simulink model "e2eDRL_ACC"  (R2023a)
settings: Solver=FixedStepAuto  StartTime=0.0  StopTime=200  FixedStep=0.1  RelTol=1e-3
values from neighbouring files (symbols this model uses):
  ap_maxmin = -3 + (0-(-4))*rand()    [Reset.m]
  beh = bernoulli_sample(prob_accp)    [Reset.m]
  dt = 0 + (2-0)*rand()    [Reset.m]    (also in Speed_replan.m = ds/v_backward(N+1-k))
  t1 = 5 + (100-5)*rand()    [Reset.m]
  Ts = 0.1    [Reset.m]
  v0_ego = 100/3.6    (= 27.7777777778)    [Reset.m]
  v0_lead = lower_bound_v0 + (upper_bound_v0-lower_bound_v0)*rand()    [Reset.m]
  v_des = sample_integer_interval(20,60,10)/3.6    [Reset.m]
  x0_ego = 0    [Reset.m]
  x0_lead = max(min(t_gap*v0_ego+D_default+5*randn(),80),15)    [Reset.m]
libraries: simulink x4
settings Model: Creator=The MathWorks, Inc.  LastModifiedBy=Administrator
settings SolverCC: AlgebraicLoopSolver=TrustRegion
settings DataIOCC: ReturnWorkspaceOutputs=off
settings DebuggingCC: UnconnectedInputMsg=warning  UnconnectedOutputMsg=warning  UnconnectedLineMsg=warning  ArithmeticOperatorsInVariantConditions=warning
settings ModelReferenceCC: EnableRefExpFcnMdlSchedulingChecks=on
settings SFSimCC: SimUseLocalCustomCode=off
settings RTWCC: RTWUseLocalCustomCode=off  DLArmComputeVersion=19.05
settings CodeAppCC: StateflowObjectComments=on

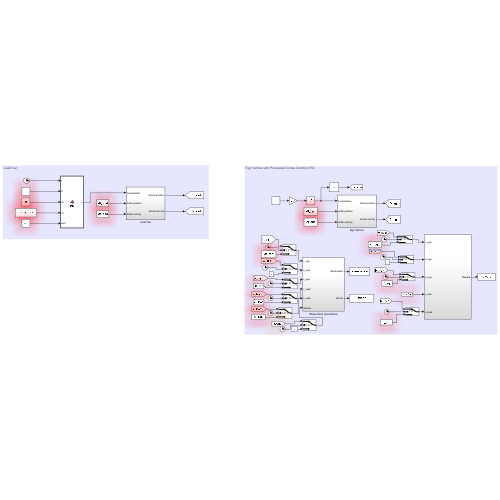
[thumbnail: Simulink's stored preview of the top-level diagram]
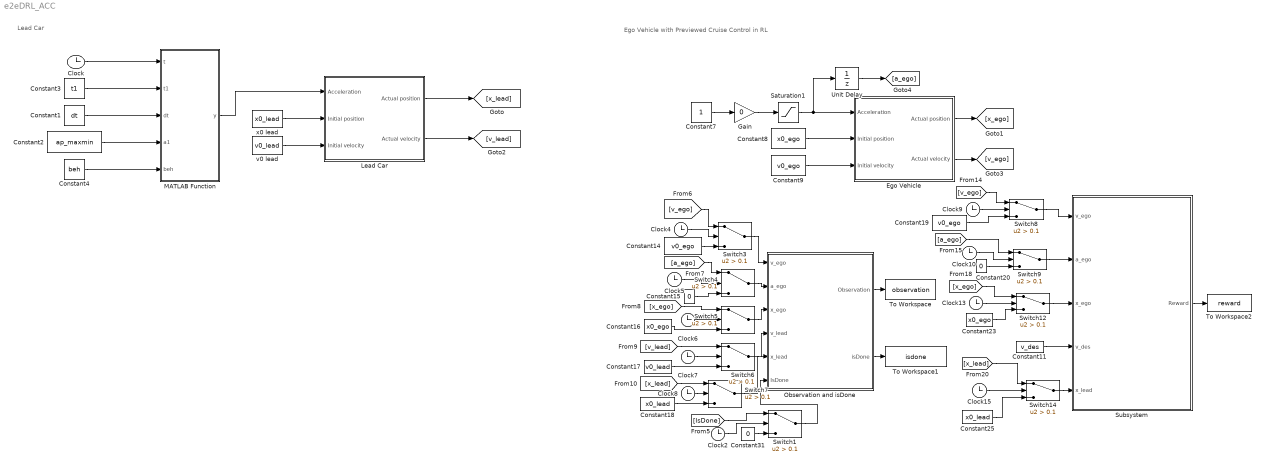
== system e2eDRL_ACC ==
  note: Lead Car
  note: Ego Vehicle with Previewed Cruise Control in RL
  Clock{,2,4..10,13,15} (11 alike) : Clock
  Constant1 : Constant  Value=dt  SampleTime=Ts
  Constant11 : Constant  Value=v_des  SampleTime=Ts
  Constant14 : Constant  Value=v0_ego  SampleTime=Ts
  Constant15 : Constant  Value=0
  Constant16 : Constant  Value=x0_ego  SampleTime=Ts
  Constant17 : Constant  Value=v0_lead  SampleTime=Ts
  Constant18 : Constant  Value=x0_lead  SampleTime=Ts
  Constant19 : Constant  Value=v0_ego  SampleTime=Ts
  Constant2 : Constant  Value=ap_maxmin  SampleTime=Ts
  Constant20 : Constant  Value=0
  Constant23 : Constant  Value=x0_ego  SampleTime=Ts
  Constant25 : Constant  Value=x0_lead  SampleTime=Ts
  Constant3 : Constant  Value=t1  SampleTime=Ts
  Constant31 : Constant  Value=0
  Constant4 : Constant  Value=beh  SampleTime=Ts
  Constant7 : Constant
  Constant8 : Constant  Value=x0_ego  SampleTime=Ts
  Constant9 : Constant  Value=v0_ego  SampleTime=Ts
  Ego Vehicle : Subsystem
  Gain : Gain  Gain=0
  Lead Car : Subsystem
  MATLAB Function : MATLAB Function  TreatAsAtomicUnit=on
  Observation and isDone : Subsystem
  Saturation1 : Saturate  UpperLimit=2  LowerLimit=-3
  Subsystem : Subsystem
  Switch{1,3..9,12,14} (10 alike) : Switch  Criteria=u2 > Threshold  Threshold=0.1  SaturateOnIntegerOverflow=off  InputSameDT=off
  To Workspace : ToWorkspace  VariableName=observation  SampleTime=-1
  To Workspace1 : ToWorkspace  VariableName=isdone  SampleTime=-1
  To Workspace2 : ToWorkspace  VariableName=reward  SampleTime=-1
  Unit Delay : UnitDelay  SampleTime=-1  HasFrameUpgradeWarning=on
  v0 lead : Constant  Value=v0_lead  SampleTime=Ts
  x0 lead : Constant  Value=x0_lead  SampleTime=Ts
  wires:
  x0 lead/1 -> Lead Car/2(Initial position)
  v0 lead/1 -> Lead Car/3(Initial velocity)
  Lead Car/1(Actual position) -> [x_lead]
  Clock/1 -> MATLAB Function/1(t)
  Constant1/1 -> MATLAB Function/3(dt)
  Constant2/1 -> MATLAB Function/4(a1)
  MATLAB Function/1(y) -> Lead Car/1(Acceleration)
  Constant3/1 -> MATLAB Function/2(t1)
  Constant4/1 -> MATLAB Function/5(beh)
  Constant7/1 -> Gain/1
  Gain/1 -> Saturation1/1
  Saturation1/1 -> Unit Delay/1, Ego Vehicle/1(Acceleration)
  Constant8/1 -> Ego Vehicle/2(Initial position)
  Constant9/1 -> Ego Vehicle/3(Initial velocity)
  Ego Vehicle/1(Actual position) -> [x_ego]
  Lead Car/2(Actual velocity) -> [v_lead]
  Ego Vehicle/2(Actual velocity) -> [v_ego]
  Observation and isDone/1(Observation) -> To Workspace/1
  Observation and isDone/2(isDone) -> To Workspace1/1
  Subsystem/1(Reward) -> To Workspace2/1
  Unit Delay/1 -> [a_ego]
  Constant11/1 -> Subsystem/4(v_des)
  Switch3/1 -> Observation and isDone/1(v_ego)
  [v_ego] -> Switch3/1
  Clock4/1 -> Switch3/2
  Constant14/1 -> Switch3/3
  [a_ego] -> Switch4/1
  Switch4/1 -> Observation and isDone/2(a_ego)
  Clock5/1 -> Switch4/2
  Constant15/1 -> Switch4/3
  Switch5/1 -> Observation and isDone/3(x_ego)
  [x_ego] -> Switch5/1
  Clock6/1 -> Switch5/2
  Constant16/1 -> Switch5/3
  Switch6/1 -> Observation and isDone/4(v_lead)
  [v_lead] -> Switch6/1
  Clock7/1 -> Switch6/2
  Constant17/1 -> Switch6/3
  Switch7/1 -> Observation and isDone/5(x_lead)
  [x_lead] -> Switch7/1
  Clock8/1 -> Switch7/2
  Constant18/1 -> Switch7/3
  Switch8/1 -> Subsystem/1(v_ego)
  [v_ego] -> Switch8/1
  Constant19/1 -> Switch8/3
  Clock9/1 -> Switch8/2
  Switch9/1 -> Subsystem/2(a_ego)
  [a_ego] -> Switch9/1
  Clock10/1 -> Switch9/2
  Constant20/1 -> Switch9/3
  [x_ego] -> Switch12/1
  Clock13/1 -> Switch12/2
  Constant23/1 -> Switch12/3
  Switch14/1 -> Subsystem/5(x_lead)
  [x_lead] -> Switch14/1
  Clock15/1 -> Switch14/2
  Constant25/1 -> Switch14/3
  Switch1/1 -> Observation and isDone/6(IsDone)
  [IsDone] -> Switch1/1
  Clock2/1 -> Switch1/2
  Constant31/1 -> Switch1/3
  Switch12/1 -> Subsystem/3(x_ego)

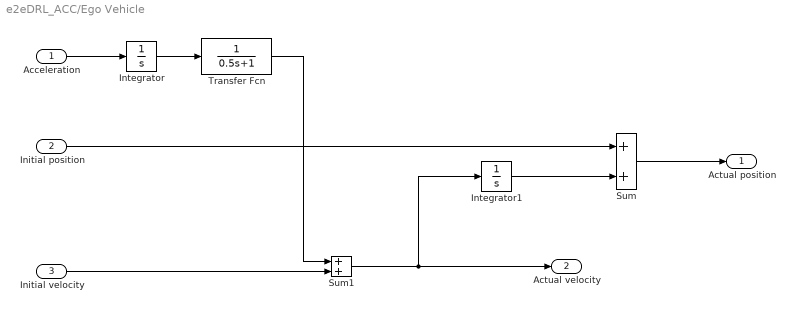
== system e2eDRL_ACC/Ego Vehicle ==
  Acceleration : Inport
  Initial position : Inport  Port=2
  Initial velocity : Inport  Port=3
  Integrator : Integrator
  Integrator1 : Integrator
  Sum : Sum
  Sum1 : Sum
  Transfer Fcn : TransferFcn  Denominator=[0.5 1]
  Actual position : Outport  VectorParamsAs1DForOutWhenUnconnected=off
  Actual velocity : Outport  Port=2  VectorParamsAs1DForOutWhenUnconnected=off
  wires:
  Transfer Fcn/1 -> Sum1/1
  Initial velocity/1 -> Sum1/2
  Sum/1 -> Actual position/1
  Integrator/1 -> Transfer Fcn/1
  Sum1/1 -> Integrator1/1, Actual velocity/1
  Acceleration/1 -> Integrator/1
  Initial position/1 -> Sum/1
  Integrator1/1 -> Sum/2

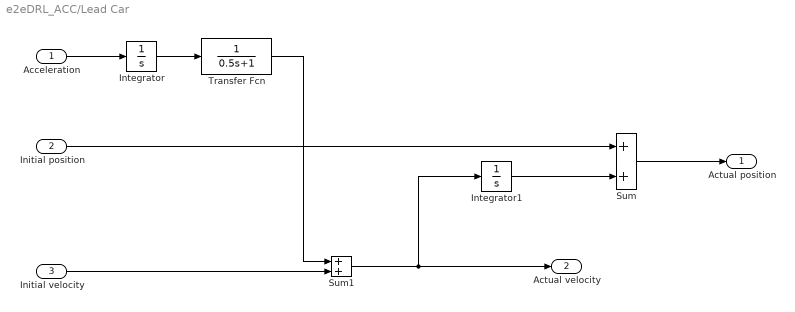
== system e2eDRL_ACC/Lead Car ==
  Acceleration : Inport
  Initial position : Inport  Port=2
  Initial velocity : Inport  Port=3
  Integrator : Integrator
  Integrator1 : Integrator
  Sum : Sum
  Sum1 : Sum
  Transfer Fcn : TransferFcn  Denominator=[0.5 1]
  Actual position : Outport  VectorParamsAs1DForOutWhenUnconnected=off
  Actual velocity : Outport  Port=2  VectorParamsAs1DForOutWhenUnconnected=off
  wires:
  Transfer Fcn/1 -> Sum1/1
  Initial velocity/1 -> Sum1/2
  Sum/1 -> Actual position/1
  Integrator/1 -> Transfer Fcn/1
  Sum1/1 -> Integrator1/1, Actual velocity/1
  Acceleration/1 -> Integrator/1
  Initial position/1 -> Sum/1
  Integrator1/1 -> Sum/2

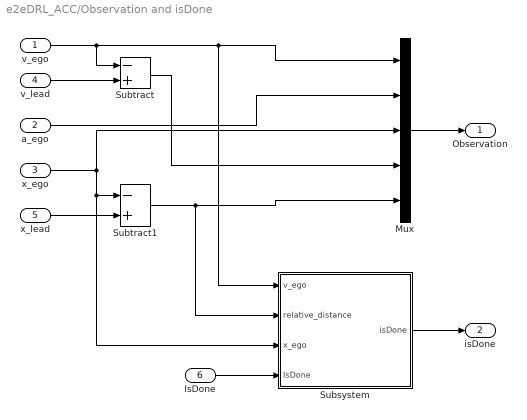
== system e2eDRL_ACC/Observation and isDone ==
  v_ego : Inport
  a_ego : Inport  Port=2
  x_ego : Inport  Port=3
  v_lead : Inport  Port=4
  x_lead : Inport  Port=5
  IsDone : Inport  Port=6
  Mux : Mux  Inputs=5
  Subsystem : Subsystem
  Subtract : Sum  Inputs=-+
  Subtract1 : Sum  Inputs=-+
  Observation : Outport
  isDone : Outport  Port=2
  wires:
  Mux/1 -> Observation/1
  v_ego/1 -> Subsystem/1(v_ego), Mux/1, Subtract/1
  v_lead/1 -> Subtract/2
  a_ego/1 -> Mux/2
  x_ego/1 -> Mux/3, Subsystem/3(x_ego), Subtract1/1
  x_lead/1 -> Subtract1/2
  Subtract1/1 -> Subsystem/2(relative_distance), Mux/5
  Subtract/1 -> Mux/4
  Subsystem/1(isDone) -> isDone/1
  IsDone/1 -> Subsystem/4(IsDone)

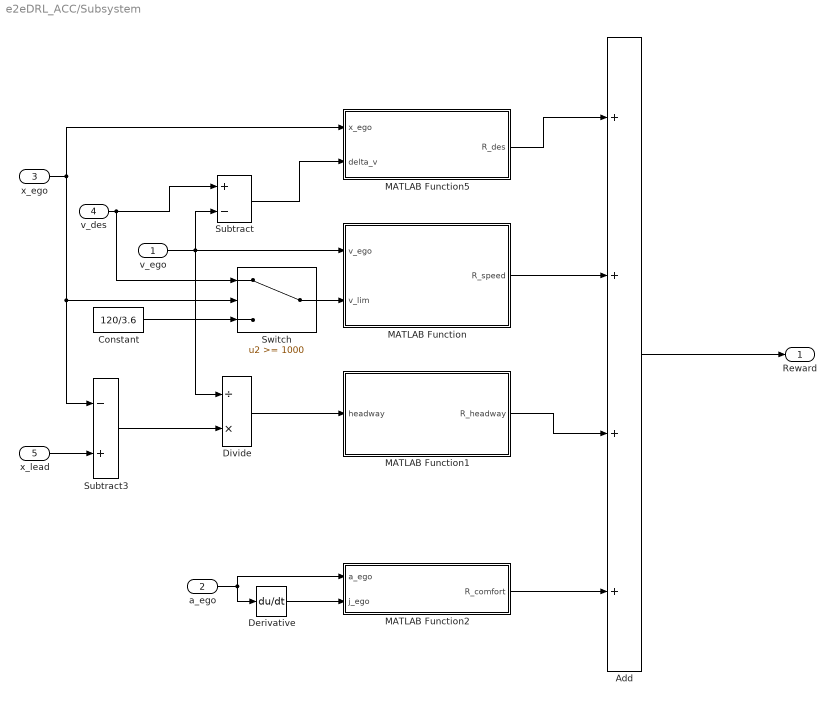
== system e2eDRL_ACC/Subsystem ==
  v_ego : Inport
  a_ego : Inport  Port=2
  x_ego : Inport  Port=3
  v_des : Inport  Port=4
  x_lead : Inport  Port=5
  Add : Sum  Inputs=++++
  Constant : Constant  Value=120/3.6
  Derivative : Derivative
  Divide : Product  Inputs=/*
  MATLAB Function : MATLAB Function  TreatAsAtomicUnit=on
  MATLAB Function1 : MATLAB Function  TreatAsAtomicUnit=on
  MATLAB Function2 : MATLAB Function  TreatAsAtomicUnit=on
  MATLAB Function5 : MATLAB Function  TreatAsAtomicUnit=on
  Subtract : Sum  Inputs=+-
  Subtract3 : Sum  Inputs=-+
  Switch : Switch  Threshold=1000  SaturateOnIntegerOverflow=off  InputSameDT=off
  Reward : Outport
  wires:
  x_lead/1 -> Subtract3/2
  v_ego/1 -> Divide/1, MATLAB Function/1(v_ego), Subtract/2
  Subtract3/1 -> Divide/2
  Divide/1 -> MATLAB Function1/1(headway)
  v_des/1 -> Switch/1, Subtract/1
  x_ego/1 -> MATLAB Function5/1(x_ego), Switch/2, Subtract3/1
  Add/1 -> Reward/1
  MATLAB Function5/1(R_des) -> Add/1
  MATLAB Function/1(R_speed) -> Add/2
  MATLAB Function1/1(R_headway) -> Add/3
  MATLAB Function2/1(R_comfort) -> Add/4
  a_ego/1 -> Derivative/1, MATLAB Function2/1(a_ego)
  Derivative/1 -> MATLAB Function2/2(j_ego)
  Subtract/1 -> MATLAB Function5/2(delta_v)
  Switch/1 -> MATLAB Function/2(v_lim)
  Constant/1 -> Switch/3

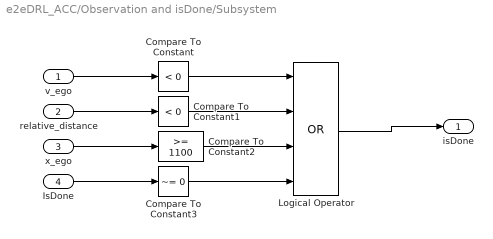
== system e2eDRL_ACC/Observation and isDone/Subsystem ==
  v_ego : Inport
  relative_distance : Inport  Port=2
  x_ego : Inport  Port=3
  IsDone : Inport  Port=4
  Compare To Constant : simulink/Logic and Bit Operations/Compare To Constant  relop=<  const=0  OutDataTypeStr=boolean
  Compare To Constant1 : simulink/Logic and Bit Operations/Compare To Constant  relop=<  const=0  OutDataTypeStr=boolean
  Compare To Constant2 : simulink/Logic and Bit Operations/Compare To Constant  relop=>=  const=1100  OutDataTypeStr=boolean
  Compare To Constant3 : simulink/Logic and Bit Operations/Compare To Constant  relop=~=  const=0  OutDataTypeStr=boolean
  Logical Operator : Logic  Operator=OR  Inputs=4  AllPortsSameDT=off  OutDataTypeStr=boolean
  isDone : Outport
  wires:
  v_ego/1 -> Compare To Constant/1
  relative_distance/1 -> Compare To Constant1/1
  x_ego/1 -> Compare To Constant2/1
  Compare To Constant2/1 -> Logical Operator/3
  Compare To Constant1/1 -> Logical Operator/2
  Compare To Constant/1 -> Logical Operator/1
  Logical Operator/1 -> isDone/1
  IsDone/1 -> Compare To Constant3/1
  Compare To Constant3/1 -> Logical Operator/4

== matlab function e2eDRL_ACC/MATLAB Function ==
  data: t input; t1 input; y output; dt input; a1 input; beh input
function y = fcn(t,t1,dt,a1,beh)
if beh==0
    j1=2;
    j2=-1.5;
    if t<t1
        y=0;
    elseif t<t1+a1/j1
        y=j1*(t-t1);
    elseif t<t1+a1/j1+dt
        y=a1;
    elseif t<t1+a1/j1+dt-a1/j2
        y=a1+j2*(t-t1-a1/j1-dt);
    else
        y=0;
    end
else
    j1=-1.5;
    j2=2;
    if t<t1
        y=0;
    elseif t<t1+a1/j1
        y=j1*(t-t1);
    elseif t<t1+a1/j1+dt
        y=a1;
    elseif t<t1+a1/j1+dt-a1/j2
        y=a1+j2*(t-t1-a1/j1-dt);
    else
        y=0;
    end
end

== matlab function e2eDRL_ACC/Subsystem/MATLAB Function ==
  data: v_ego input; R_speed output; v_lim input
function R_speed = fcn(v_ego,v_lim)
R_speed=v_lim-max(0,v_lim-v_ego);

== matlab function e2eDRL_ACC/Subsystem/MATLAB Function1 ==
  data: headway input; R_headway output
function R_headway = fcn(headway)
if headway <= 0
    R_headway = -1000;
elseif headway <= 1.4
    R_headway = -1000 + 1000/1.4*sqrt(1.4^2-(headway-1.4)^2);
else
    R_headway = 0;
end
end

== matlab function e2eDRL_ACC/Subsystem/MATLAB Function2 ==
  data: a_ego input; j_ego input; R_comfort output
function R_comfort = fcn(a_ego,j_ego)
R_comfort = -a_ego^2-j_ego^2;

== matlab function e2eDRL_ACC/Subsystem/MATLAB Function5 ==
  data: x_ego input; R_des output; delta_v input
function R_des = fcn(x_ego,delta_v)
if x_ego >= 1000
    if delta_v <= -1
        R_des = -500;
    elseif delta_v < 0
        R_des = 500*delta_v;
    elseif delta_v <= 1
        R_des = 1000*sqrt(1-delta_v^2);
    else
        R_des = 0;
    end
elseif x_ego >= 500 
    R_des = x_ego/2+250;
else
    R_des = x_ego;
end
